simulink model "Q2_a_3"  (R2022a)
settings: Solver=ode15s  StartTime=0.0  StopTime=20  RelTol=1e-3
settings Model: Creator=bhara  LastModifiedBy=manan
settings SolverCC: AlgebraicLoopSolver=TrustRegion
settings DebuggingCC: UnconnectedInputMsg=warning  UnconnectedOutputMsg=warning  UnconnectedLineMsg=warning  SFMachineParentedDataDiag=warning
settings RTWCC: DLArmComputeVersion=19.05

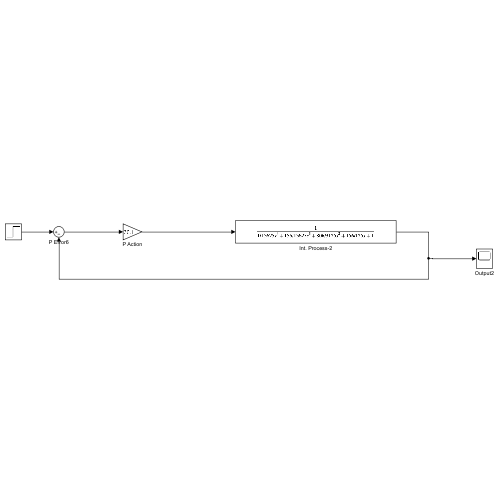
[thumbnail: Simulink's stored preview of the top-level diagram]
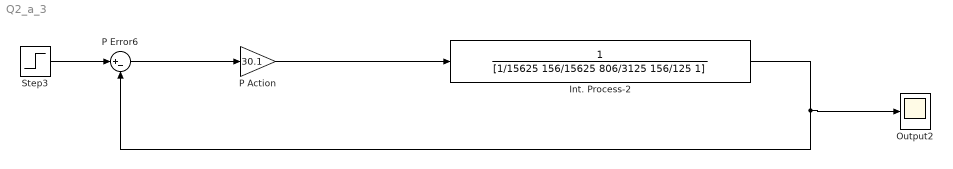
== system Q2_a_3 ==
  Int. Process-2 : TransferFcn  Denominator=[1/15625 156/15625 806/3125 156/125 1]
  Output2 : Scope
  P Action : Gain  Gain=30.1
  P Error6 : Sum  Inputs=|+-
  Step3 : Step  SampleTime=0
  wires:
  P Error6/1 -> P Action/1
  Step3/1 -> P Error6/1
  Int. Process-2/1 -> P Error6/2, Output2/1
  P Action/1 -> Int. Process-2/1
